simulink model "part3"  (R2020a)
settings: Solver=VariableStepAuto  StartTime=0.0  StopTime=86400*5  RelTol=1e-3
values from neighbouring files (symbols this model uses):
  A = [0              1                   0       0 ... (first row only)    [p4.m]    (also in part3.m)
  B = [ 0             0 ... (first row only)    [p4.m]    (also in part3.m)
  C = [1/r_0      0       0       0 ... (first row only)    [p4.m]    (also in part3.m)
  T0 = 86400    [part3.m]
  xo = [r_0 0 0 0]    [part3.m]
settings Model: Creator=mimshin  LastModifiedBy=Edwin

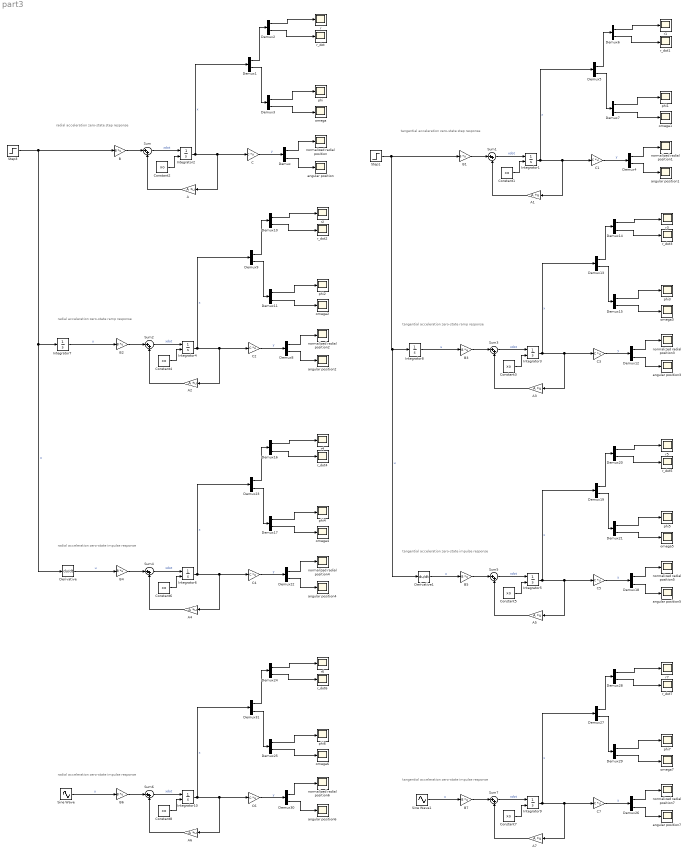
== system part3 ==
  note: radial acceleration zero-state step response
  note: tangential acceleration zero-state step response
  note: radial acceleration zero-state ramp response
  note: tangential acceleration zero-state ramp response
  note: tangential acceleration zero-state impulse response
  note: radial acceleration zero-state impulse response
  note: radial acceleration zero-state impulse response
  note: tangential acceleration zero-state impulse response
  A{,1..7} (8 alike) : Gain  Gain=A  Multiplication=Matrix(K*u)
  B{,1..7} (8 alike) : Gain  Gain=B  Multiplication=Matrix(K*u)
  C{,1..7} (8 alike) : Gain  Gain=C  Multiplication=Matrix(K*u)
  Constant{1..8} (8 alike) : Constant  Value=xo
  Demux{,1..31} (32 alike) : Demux  Outputs=2
  Derivative : Derivative
  Derivative1 : Derivative
  Integrator{1..6,9..10} (8 alike) : Integrator  InitialConditionSource=external  InitialCondition=[0; 0; 0; 0]
  Integrator7 : Integrator  InitialCondition=[0; 0]
  Integrator8 : Integrator  InitialCondition=[0; 0]
  Sine Wave : Sin  Amplitude=[1; 0]  Frequency=[1/T0; 0]  SampleTime=0  VectorParams1D=off
  Sine Wave1 : Sin  Amplitude=[0; 1]  Frequency=[0; 1/T0]  SampleTime=0  VectorParams1D=off
  Step1 : Step  Before=[0;0]  After=[0; 1]  SampleTime=0  VectorParams1D=off
  Step3 : Step  Before=[0;0]  After=[1; 0]  SampleTime=0  VectorParams1D=off
  Sum{,1..7} (8 alike) : Sum  Inputs=|++
  angular position{,1..7} (8 alike) : Scope
  normalized radial position{,1..7} (8 alike) : Scope
  omega{,1..7} (8 alike) : Scope
  phi{,1..7} (8 alike) : Scope
  r{,1..7} (8 alike) : Scope
  r_dot{,1..7} (8 alike) : Scope
  wires:
  C/1 -> Demux/1  "y"
  Sum/1 -> Integrator2/1  "xdot"
  A/1 -> Sum/2
  Integrator2/1 -> Demux1/1, C/1, A/1  "x"
  B/1 -> Sum/1
  Demux/1 -> normalized radial position/1
  Demux/2 -> angular position/1
  Constant2/1 -> Integrator2/2
  Demux1/1 -> Demux2/1
  Demux1/2 -> Demux3/1
  Demux2/1 -> r/1
  Demux2/2 -> r_dot/1
  Demux3/1 -> phi/1
  Demux3/2 -> omega/1
  Demux6/2 -> r_dot1/1
  Demux5/2 -> Demux7/1
  Constant1/1 -> Integrator1/2
  Demux5/1 -> Demux6/1
  Demux6/1 -> r1/1
  Demux7/1 -> phi1/1
  Demux7/2 -> omega1/1
  Demux4/1 -> normalized radial position1/1
  Demux4/2 -> angular position1/1
  A1/1 -> Sum1/2
  Integrator1/1 -> Demux5/1, C1/1, A1/1  "x"
  Sum1/1 -> Integrator1/1  "xdot"
  C1/1 -> Demux4/1  "y"
  B1/1 -> Sum1/1
  Demux10/2 -> r_dot2/1
  Demux9/2 -> Demux11/1
  Constant4/1 -> Integrator4/2
  Demux10/1 -> r2/1
  Demux11/1 -> phi2/1
  Integrator7/1 -> B2/1  "u"
  B3/1 -> Sum3/1
  C3/1 -> Demux12/1  "y"
  A3/1 -> Sum3/2
  Integrator3/1 -> Demux13/1, C3/1, A3/1  "x"
  Demux12/1 -> normalized radial position3/1
  Demux11/2 -> omega2/1
  Demux12/2 -> angular position3/1
  Sum3/1 -> Integrator3/1  "xdot"
  Demux15/2 -> omega3/1
  Integrator8/1 -> B3/1  "u"
  Demux15/1 -> phi3/1
  Demux14/1 -> r3/1
  Demux9/1 -> Demux10/1
  Constant3/1 -> Integrator3/2
  Demux14/2 -> r_dot3/1
  Demux13/2 -> Demux15/1
  Demux8/1 -> normalized radial position2/1
  Demux8/2 -> angular position2/1
  A2/1 -> Sum2/2
  Integrator4/1 -> Demux9/1, C2/1, A2/1  "x"
  Sum2/1 -> Integrator4/1  "xdot"
  C2/1 -> Demux8/1  "y"
  Demux13/1 -> Demux14/1
  B2/1 -> Sum2/1
  B4/1 -> Sum4/1
  Demux19/1 -> Demux20/1
  Sum4/1 -> Integrator6/1  "xdot"
  Integrator6/1 -> Demux23/1, C4/1, A4/1  "x"
  Demux22/2 -> angular position4/1
  Demux20/2 -> r_dot5/1
  Sum5/1 -> Integrator5/1  "xdot"
  Constant5/1 -> Integrator5/2
  A4/1 -> Sum4/2
  Demux20/1 -> r5/1
  Demux22/1 -> normalized radial position4/1
  Demux23/1 -> Demux16/1
  Demux21/1 -> phi5/1
  Demux21/2 -> omega5/1
  Demux18/2 -> angular position5/1
  Demux18/1 -> normalized radial position5/1
  Integrator5/1 -> Demux19/1, C5/1, A5/1  "x"
  Demux17/2 -> omega4/1
  C5/1 -> Demux18/1  "y"
  B5/1 -> Sum5/1
  Demux17/1 -> phi4/1
  A5/1 -> Sum5/2
  Constant6/1 -> Integrator6/2
  Demux19/2 -> Demux21/1
  Demux23/2 -> Demux17/1
  Demux16/2 -> r_dot4/1
  Derivative/1 -> B4/1  "u"
  C4/1 -> Demux22/1  "y"
  Demux16/1 -> r4/1
  Step3/1 -> Integrator7/1, Derivative/1, B/1  "u"
  Step1/1 -> Derivative1/1, Integrator8/1, B1/1  "u"
  Derivative1/1 -> B5/1  "u"
  Demux24/1 -> r6/1
  C6/1 -> Demux30/1  "y"
  Demux31/2 -> Demux25/1
  Demux24/2 -> r_dot6/1
  Demux27/2 -> Demux29/1
  Demux25/1 -> phi6/1
  A7/1 -> Sum7/2
  Demux25/2 -> omega6/1
  C7/1 -> Demux26/1  "y"
  Demux26/1 -> normalized radial position7/1
  Demux26/2 -> angular position7/1
  Integrator9/1 -> Demux27/1, C7/1, A7/1  "x"
  Demux29/2 -> omega7/1
  Demux29/1 -> phi7/1
  Demux31/1 -> Demux24/1
  Constant7/1 -> Integrator9/2
  A6/1 -> Sum6/2
  Demux30/1 -> normalized radial position6/1
  B7/1 -> Sum7/1
  Demux30/2 -> angular position6/1
  Sum7/1 -> Integrator9/1  "xdot"
  Constant8/1 -> Integrator10/2
  Demux28/2 -> r_dot7/1
  Demux27/1 -> Demux28/1
  Demux28/1 -> r7/1
  Sum6/1 -> Integrator10/1  "xdot"
  Integrator10/1 -> Demux31/1, C6/1, A6/1  "x"
  B6/1 -> Sum6/1
  Sine Wave/1 -> B6/1  "u"
  Sine Wave1/1 -> B7/1  "u"
